simulink model "heli_master_2015b"  (R2015b)
settings: Solver=ode1  SolverMode=SingleTasking  StartTime=0.0  StopTime=inf  FixedStep=0.002  RelTol=1e-3
PostLoadFcn:
  | qc_set_target_type(getConfigSet(bdroot, 'QUARC Default Target Configuration'));
values from neighbouring files (symbols this model uses):
  K = P_predicted * C' * inv(C * P_predicted * C' + obj.W)    [ExtendedKalmanFilter.m]    (also in HighGainObserver.m = zeros(8, 2); StateFeedback.m = zeros(2, 6))
  lamb = block.ContStates.Data(3)    [BetterSimulation.m]    (also in FeedbackLinearization.m = x(3); dyn_ext_eps_meas.mat = [0 0 0 0 0 0 0 0 0 0 0 0 ... (30000 elements, 6000x5)]; e_-10_10_l_0_120_t_10.mat = [0 3.40359280049e-12 1.08295188827e-10 8.177826625e-10 3.426; e_-10_10_l_0_120_t_20.mat = [0 1.06295178385e-13 3.38915391498e-12 2.56636695446e-11 1.0)
  phi = block.ContStates.Data(1)    [BetterSimulation.m]    (also in FeedbackLinearization.m = x(1); dyn_ext_eps_meas.mat = [0 0 0 0 0 0 0 0 0 0 0 0 ... (18000 elements, 6000x3)]; e_-10_10_l_0_120_t_10.mat = [3.57789727367e-14 3.32260230971e-07 2.63920782562e-06 8.843; e_-10_10_l_0_120_t_20.mat = [3.52494450884e-15 1.04005854531e-08 8.29611824462e-08 2.791)
  R = diag(R_diag)    [compute_lqr_feedback.m]    (also in first_tvlqr_test.mat = [1  0; 0  1])
  vb = block.InputPort(2).Data    [BetterSimulation.m]    (also in analyze_eps_meas.m = [log_neg.signals(2).values; log_pos.signals(2).values]; dyn_ext_eps_meas.mat = [2.46662433384 2.46662437608 2.46662467016 2.46662546356 2.4; e_-10_10_l_0_120_t_10.mat = [3.03305943788 3.0306076999 3.02819113358 3.02581096907 3.02; e_-10_10_l_0_120_t_20.mat = [3.03305943788 3.0329822422 3.03290486178 3.03282733913 3.03)
  vf = block.InputPort(1).Data    [BetterSimulation.m]    (also in analyze_eps_meas.m = [log_neg.signals(1).values; log_pos.signals(1).values]; dyn_ext_eps_meas.mat = [2.46662433384 2.46662437608 2.46662467016 2.46662546356 2.4; e_-10_10_l_0_120_t_10.mat = [3.03305943788 3.03551133878 3.03792903521 3.04031223633 3.0; e_-10_10_l_0_120_t_20.mat = [3.03305943788 3.03313663866 3.03321405463 3.03329167331 3.0)
undefined symbols (not defined in the file or in its folder): HIL, qc_get_step_size
libraries: simulink_extras x25, quarc_library x4
(part 1 of 2)
settings Model: SimulationMode=external  ExtModeTrigDuration=120000  ExtModeTrigLevel=0.500000  Creator=Rchan  LastModifiedBy=robertph
settings SolverCC: PositivePriorityOrder=on
settings DataIOCC: SaveFormat=Array
settings OptimizationCC: ExpressionDepthLimit=2147483647  InitFltsAndDblsToZero=on
settings DebuggingCC: SaveWithParameterizedLinksMsg=none  UnderspecifiedInitializationDetection=Classic  MergeDetectMultiDrivingBlocksExec=none  SolverPrmCheckMsg=warning  MultiTaskDSMMsg=warning  FcnCallInpInsideContextMsg=EnableAllAsWarning  AllowSymbolicDim=on  StateNameClashWarn=warning
settings HardwareCC: ProdBitPerPointer=32  ProdLargestAtomicFloat=None  ProdIntDivRoundTo=Undefined  ProdEndianess=Unspecified  ProdWordSize=32  ProdHWDeviceType=32-bit Generic
settings RTWCC: SystemTargetFile=quarc_win64.tlc  TemplateMakefile=quarc_default_tmf  Description=QUARC Win64 Target
settings GRTTargetCC: ParMdlRefBuildCompliant=off  CompOptLevelCompliant=off  GeneratePreprocessorConditionals=Disable all  CombineOutputUpdateFcns=off  MatFileLogging=off  GRTInterface=on  UseToolchainInfoCompliant=off  ExtMode=on  ExtModeMexFile=quarc_comm
settings ConfigComp: CovModelRefEnable=Off  CovSFcnEnable=off

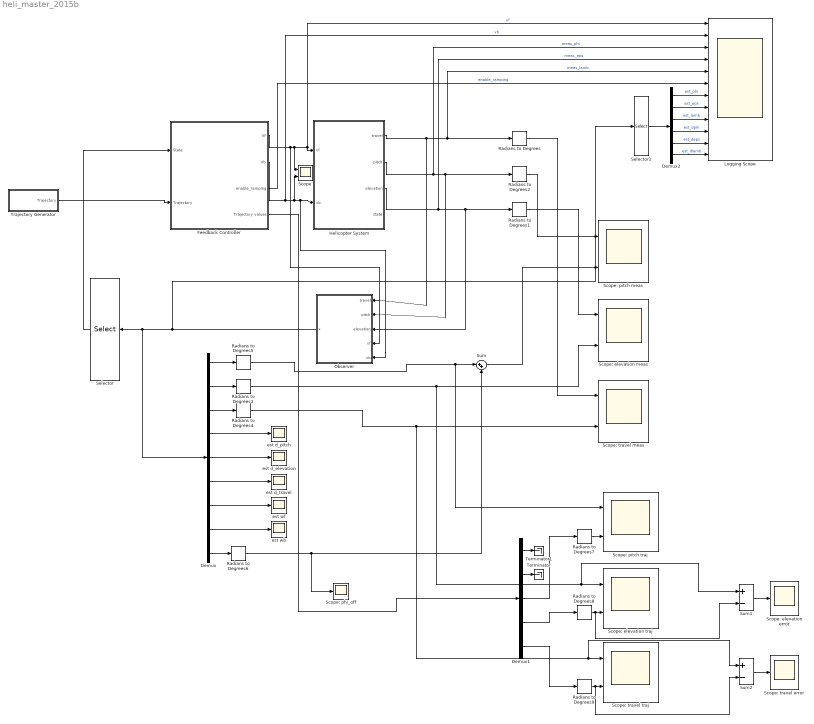
== system heli_master_2015b ==
  Demux : Demux  Outputs=9
  Demux1 : Demux  Outputs=5
  Demux2 : Demux  Outputs=6
  Feedback Controller : Subsystem
  Helicopter System : Subsystem  Variant=on  OverrideUsingVariant=HiL
  Logging Scope : Scope  NumInputPorts=12
  Observer : Subsystem
  Radians to Degrees{,1..9} (10 alike) : simulink_extras/Transformations/Radians to Degrees
  Scope : Scope  NumInputPorts=2
  Scope: elevation error : Scope
  Scope: elevation meas : Scope  NumInputPorts=2
  Scope: elevation traj : Scope  NumInputPorts=2
  Scope: phi_off : Scope
  Scope: pitch meas : Scope  NumInputPorts=2
  Scope: pitch traj : Scope  NumInputPorts=2
  Scope: travel error : Scope
  Scope: travel meas : Scope  NumInputPorts=2
  Scope: travel traj : Scope  NumInputPorts=2
  Selector : Selector  InputPortWidth=9  IndexOptions=Index vector (dialog)  Indices=[1 2 3 4 5 6 7 8]  OutputSizes=1
  Selector1 : Selector  InputPortWidth=9  IndexOptions=Index vector (dialog)  Indices=[1 2 3 4 5 6]  OutputSizes=1
  Sum : Sum  Inputs=|++
  Sum1 : Sum  Inputs=+-
  Sum2 : Sum  Inputs=+-
  Terminator : Terminator
  Terminator1 : Terminator
  Trajectory Generator : Subsystem
  est d_elevation : Scope
  est d_pitch : Scope
  est d_travel : Scope
  est wb : Scope
  est wf : Scope
  wires:
  Helicopter System/1(travel) -> Observer/1(travel), Logging Scope/5, Radians to Degrees/1  "meas_lamb"
  Helicopter System/3(elevation) -> Logging Scope/4, Observer/3(elevation), Radians to Degrees1/1  "meas_eps"
  Helicopter System/2(pitch) -> Logging Scope/3, Observer/2(pitch), Radians to Degrees2/1  "meas_phi"
  Radians to Degrees/1 -> Scope: travel meas/1
  Radians to Degrees2/1 -> Scope: pitch meas/1
  Radians to Degrees1/1 -> Scope: elevation meas/1
  Feedback Controller/2(Vb) -> Logging Scope/2, Scope/2, Observer/5(vb), Helicopter System/2(vb)  "vb"
  Feedback Controller/1(Vf) -> Observer/4(vf), Scope/1, Logging Scope/1, Helicopter System/1(vf)  "vf"
  Observer/1(x) -> Selector1/1, Selector/1, Demux/1
  Trajectory Generator/1(Trajectory) -> Feedback Controller/2(Trajectory)
  Demux/1 -> Radians to Degrees5/1
  Radians to Degrees3/1 -> Sum1/1, Scope: elevation traj/1, Scope: elevation meas/2
  Radians to Degrees4/1 -> Sum2/1, Scope: travel traj/1, Scope: travel meas/2
  Demux/2 -> Radians to Degrees3/1
  Demux/3 -> Radians to Degrees4/1
  Demux/4 -> est d_pitch/1
  Demux/5 -> est d_elevation/1
  Demux/6 -> est d_travel/1
  Demux/7 -> est wf/1
  Demux/8 -> est wb/1
  Demux/9 -> Radians to Degrees6/1
  Radians to Degrees5/1 -> Scope: pitch traj/1, Sum/1
  Sum/1 -> Scope: pitch meas/2
  Radians to Degrees6/1 -> Scope: phi_off/1, Sum/2
  Feedback Controller/3(enable_ramping) -> Logging Scope/6  "enable_ramping"
  Selector/1 -> Feedback Controller/1(State)
  Demux1/3 -> Radians to Degrees7/1
  Radians to Degrees7/1 -> Scope: pitch traj/2
  Radians to Degrees8/1 -> Sum1/2, Scope: elevation traj/2
  Radians to Degrees9/1 -> Sum2/2, Scope: travel traj/2
  Feedback Controller/4(Trajectory values) -> Demux1/1
  Demux1/4 -> Radians to Degrees8/1
  Demux1/5 -> Radians to Degrees9/1
  Demux1/2 -> Terminator/1
  Demux1/1 -> Terminator1/1
  Sum1/1 -> Scope: elevation error/1
  Sum2/1 -> Scope: travel error/1
  Selector1/1 -> Demux2/1
  Demux2/1 -> Logging Scope/7  "est_phi"
  Demux2/2 -> Logging Scope/8  "est_eps"
  Demux2/3 -> Logging Scope/9  "est_lamb"
  Demux2/4 -> Logging Scope/10  "est_dphi"
  Demux2/5 -> Logging Scope/11  "est_deps"
  Demux2/6 -> Logging Scope/12  "est_dlamb"

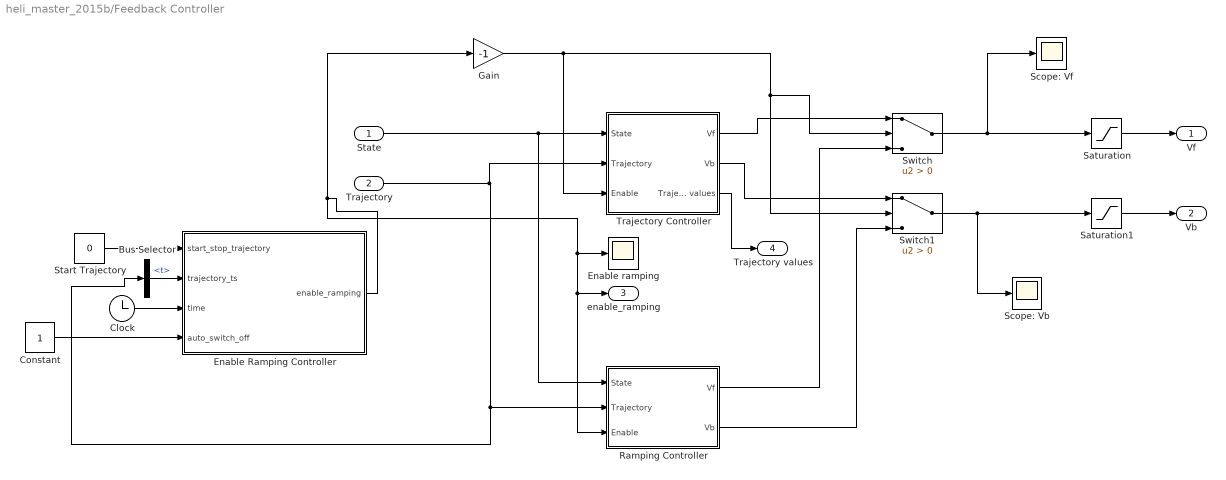
== system heli_master_2015b/Feedback Controller ==
  State : Inport
  Trajectory : Inport  Port=2
  Bus Selector : BusSelector  OutputSignals=t
  Clock : Clock
  Constant : Constant
  Enable Ramping Controller : MATLAB Function  TreatAsAtomicUnit=on
  Enable ramping : Scope
  Gain : Gain  Gain=-1
  Ramping Controller : Subsystem  mask(Ramping PID controller){ramp_period=0.1, deps_op=5, dlamb_op=10}
      mask prompts: ramp_period "Ramp period (s)"; deps_op "Elevation rate (deg/s)"; dlamb_op "Travel rate (deg/s)"
      mask help: Stabilizes an operating point, target is slowly ramped to set values.
  Saturation : Saturate  UpperLimit=5  LowerLimit=-5
  Saturation1 : Saturate  UpperLimit=5  LowerLimit=-5
  Scope: Vb : Scope
  Scope: Vf : Scope
  Start Trajectory : Constant  Value=0
  Switch : Switch  Criteria=u2 > Threshold
  Switch1 : Switch  Criteria=u2 > Threshold
  Trajectory Controller : Subsystem
  Vf : Outport
  Vb : Outport  Port=2
  enable_ramping : Outport  Port=3
  Trajectory values : Outport  Port=4
  wires:
  State/1 -> Ramping Controller/1(State), Trajectory Controller/1(State)
  Trajectory/1 -> Trajectory Controller/2(Trajectory), Bus Selector/1, Ramping Controller/2(Trajectory)
  Ramping Controller/1(Vf) -> Switch/3
  Ramping Controller/2(Vb) -> Switch1/3
  Start Trajectory/1 -> Enable Ramping Controller/1(start_stop_trajectory)
  Gain/1 -> Trajectory Controller/3(Enable), Switch1/2, Switch/2
  Switch/1 -> Saturation/1, Scope: Vf/1
  Switch1/1 -> Saturation1/1, Scope: Vb/1
  Trajectory Controller/1(Vf) -> Switch/1
  Trajectory Controller/2(Vb) -> Switch1/1
  Bus Selector/1 -> Enable Ramping Controller/2(trajectory_ts)  "<t>"
  Clock/1 -> Enable Ramping Controller/3(time)
  Saturation/1 -> Vf/1
  Saturation1/1 -> Vb/1
  Constant/1 -> Enable Ramping Controller/4(auto_switch_off)
  Enable Ramping Controller/1(enable_ramping) -> Enable ramping/1, enable_ramping/1, Ramping Controller/3(Enable), Gain/1
  Trajectory Controller/3(Trajectory values) -> Trajectory values/1

== system heli_master_2015b/Helicopter System ==
  note: 1) Add Subsystem or Model blocks as valid variant choices.
      | 2) You cannot connect blocks at this level. At simulation, connectivity is automatically
      | determined, based on the active variant and port name matching.
  vf : Inport
  vb : Inport  Port=2
  Helicopter Simulation : Subsystem  VariantControl=BetterSim  mask{ang0=[0, -20, 0], dang0=[0, 0, 0], w0=[0, 0]}
      mask prompts: ang0 "Pitch, Elevation, Travel (deg)"; dang0 "Angular velocities (deg/s)"; w0 "Rotor velocities"
      mask DialogControl DescTextVar Prompt: Simulates the helicopter system based on the equations of motion specified in system_f.m
  HiL : Subsystem  VariantControl=HiL
  Simple Simulation : Subsystem  VariantControl=SimpleSim
  Simulation with dynamic extension : Subsystem  VariantControl=DynamicExtensionSim
  travel : Outport
  pitch : Outport  Port=2
  elevation : Outport  Port=3
  state : Outport  Port=4

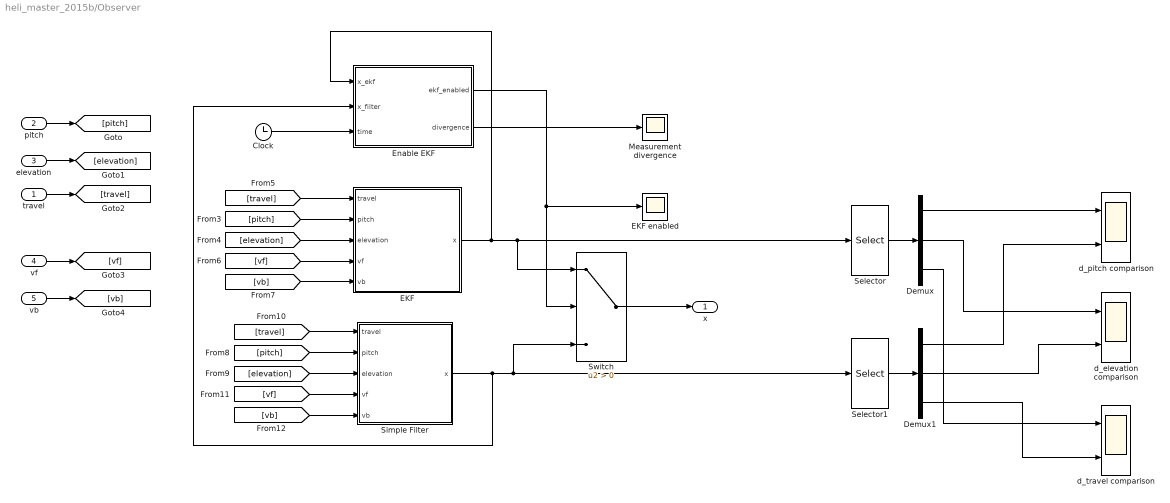
== system heli_master_2015b/Observer ==
  travel : Inport  PortDimensions=1
  pitch : Inport  Port=2  PortDimensions=1
  elevation : Inport  Port=3  PortDimensions=1
  vf : Inport  Port=4  PortDimensions=1
  vb : Inport  Port=5  PortDimensions=1
  Clock : Clock
  Demux : Demux  Outputs=3
  Demux1 : Demux  Outputs=3
  EKF : Subsystem  VariantControl=EKF
  EKF enabled : Scope
  Enable EKF : MATLAB Function  TreatAsAtomicUnit=on
  Measurement divergence : Scope
  Selector : Selector  InputPortWidth=9  IndexOptions=Index vector (dialog)  Indices=[4 5 6]  OutputSizes=1
  Selector1 : Selector  InputPortWidth=9  IndexOptions=Index vector (dialog)  Indices=[4 5 6]  OutputSizes=1
  Simple Filter : Subsystem  VariantControl=SimpleFilter
  Switch : Switch  Criteria=u2 > Threshold
  d_elevation comparison : Scope  NumInputPorts=2
  d_pitch comparison : Scope  NumInputPorts=2
  d_travel comparison : Scope  NumInputPorts=2
  x : Outport
  wires:
  Switch/1 -> x/1
  EKF/1(x) -> Enable EKF/1(x_ekf), Selector/1, Switch/1
  Simple Filter/1(x) -> Enable EKF/2(x_filter), Selector1/1, Switch/3
  Enable EKF/1(ekf_enabled) -> EKF enabled/1, Switch/2
  pitch/1 -> [pitch]
  vb/1 -> [vb]
  vf/1 -> [vf]
  travel/1 -> [travel]
  elevation/1 -> [elevation]
  [travel] -> EKF/1(travel)
  [elevation] -> EKF/3(elevation)
  [pitch] -> EKF/2(pitch)
  [vb] -> EKF/5(vb)
  [vf] -> EKF/4(vf)
  [travel] -> Simple Filter/1(travel)
  [elevation] -> Simple Filter/3(elevation)
  [pitch] -> Simple Filter/2(pitch)
  [vb] -> Simple Filter/5(vb)
  [vf] -> Simple Filter/4(vf)
  Clock/1 -> Enable EKF/3(time)
  Enable EKF/2(divergence) -> Measurement divergence/1
  Selector/1 -> Demux/1
  Selector1/1 -> Demux1/1
  Demux/1 -> d_pitch comparison/1
  Demux1/1 -> d_pitch comparison/2
  Demux/2 -> d_elevation comparison/1
  Demux1/2 -> d_elevation comparison/2
  Demux/3 -> d_travel comparison/1
  Demux1/3 -> d_travel comparison/2

== system heli_master_2015b/Trajectory Generator ==
  Bus Creator : BusCreator  Inputs=6
  Constant : Constant  Value=t
  Constant1 : Constant  Value=phi  VectorParams1D=off
  Constant2 : Constant  Value=eps  VectorParams1D=off
  Constant3 : Constant  Value=lamb  VectorParams1D=off
  Constant4 : Constant  Value=vf  VectorParams1D=off
  Constant5 : Constant  Value=vb  VectorParams1D=off
  Trajectory : Outport
  wires:
  Constant/1 -> Bus Creator/1  "t"
  Constant5/1 -> Bus Creator/6  "vb"
  Constant4/1 -> Bus Creator/5  "vf"
  Constant3/1 -> Bus Creator/4  "lamb"
  Constant2/1 -> Bus Creator/3  "eps"
  Constant1/1 -> Bus Creator/2  "phi"
  Bus Creator/1 -> Trajectory/1

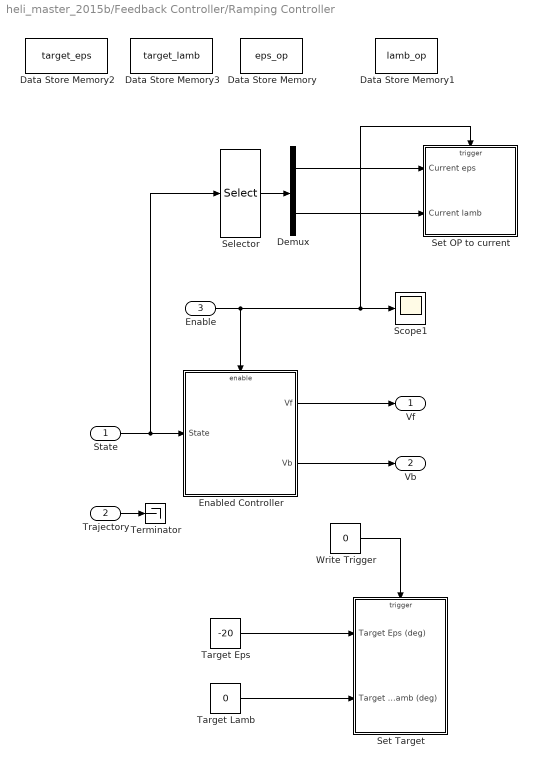
== system heli_master_2015b/Feedback Controller/Ramping Controller ==
  State : Inport
  Trajectory : Inport  Port=2
  Enable : Inport  Port=3
  Data Store Memory : DataStoreMemory  DataStoreName=eps_op  ReadBeforeWriteMsg=warning  WriteAfterWriteMsg=warning  WriteAfterReadMsg=warning  InitialValue=-29 / 180 * pi
  Data Store Memory1 : DataStoreMemory  DataStoreName=lamb_op  ReadBeforeWriteMsg=warning  WriteAfterWriteMsg=warning  WriteAfterReadMsg=warning
  Data Store Memory2 : DataStoreMemory  DataStoreName=target_eps  ReadBeforeWriteMsg=warning  WriteAfterWriteMsg=warning  WriteAfterReadMsg=warning  InitialValue=-29  OutDataTypeStr=double
  Data Store Memory3 : DataStoreMemory  DataStoreName=target_lamb  ReadBeforeWriteMsg=warning  WriteAfterWriteMsg=warning  WriteAfterReadMsg=warning  OutDataTypeStr=double
  Demux : Demux  Outputs=2
  Enabled Controller : Subsystem
  Scope1 : Scope
  Selector : Selector  InputPortWidth=8  IndexOptions=Index vector (dialog)  Indices=[2 3]  OutputSizes=1
  Set OP to current : Subsystem
  Set Target : Subsystem
  Target Eps : Constant  Value=-20
  Target Lamb : Constant  Value=0
  Terminator : Terminator
  Write Trigger : Constant  Value=0
  Vf : Outport
  Vb : Outport  Port=2
  wires:
  Enable/1 -> Scope1/1, Set OP to current/Trigger, Enabled Controller/Enable
  Demux/1 -> Set OP to current/1(Current eps)
  Demux/2 -> Set OP to current/2(Current lamb)
  State/1 -> Selector/1, Enabled Controller/1(State)
  Enabled Controller/2(Vb) -> Vb/1
  Enabled Controller/1(Vf) -> Vf/1
  Selector/1 -> Demux/1
  Target Lamb/1 -> Set Target/2(Target Lamb (deg))
  Target Eps/1 -> Set Target/1(Target Eps (deg))
  Write Trigger/1 -> Set Target/Trigger
  Trajectory/1 -> Terminator/1

== system heli_master_2015b/Feedback Controller/Trajectory Controller ==
  State : Inport
  Trajectory : Inport  Port=2
  Enable : Inport  Port=3
  Clock : Clock
  Data Store Memory : DataStoreMemory  DataStoreName=t0  ReadBeforeWriteMsg=warning  WriteAfterWriteMsg=warning  WriteAfterReadMsg=warning
  Data Store Read : DataStoreRead  Priority=10  DataStoreName=t0  SampleTime=0.002
  Enabled Controller : Subsystem
  Reset Time : Subsystem  Priority=0
  Sum : Sum  Inputs=-+|
  Vf : Outport
  Vb : Outport  Port=2
  Trajectory values : Outport  Port=3
  wires:
  Clock/1 -> Reset Time/1(Time), Sum/2
  Data Store Read/1 -> Sum/1
  Enabled Controller/1(Vf) -> Vf/1
  Enabled Controller/2(Vb) -> Vb/1
  Trajectory/1 -> Enabled Controller/3(Trajectory)
  State/1 -> Enabled Controller/2(State)
  Sum/1 -> Enabled Controller/1(Time)
  Enable/1 -> Enabled Controller/Enable, Reset Time/Trigger
  Enabled Controller/3(Trajectory values) -> Trajectory values/1

== system heli_master_2015b/Helicopter System/Helicopter Simulation ==
  vf : Inport
  vb : Inport  Port=2
  Level-2 MATLAB S-Function : M-S-Function  FunctionName=BetterSimulation  Parameters=ang0(1), ang0(2), ang0(3), dang0(1), dang0(2), dang0(3), w0(1), w0(2)
  Vector Concatenate : Concatenate  NumInputs=8
  d_elevation : Scope
  d_pitch : Scope
  d_travel : Scope
  dd_elevation : Scope
  dd_pitch : Scope
  dd_travel : Scope
  wb : Scope
  wf : Scope
  pitch : Outport
  elevation : Outport  Port=2
  travel : Outport  Port=3
  state : Outport  Port=4
  wires:
  vf/1 -> Level-2 MATLAB S-Function/1
  vb/1 -> Level-2 MATLAB S-Function/2
  Level-2 MATLAB S-Function/1 -> Vector Concatenate/1, pitch/1
  Level-2 MATLAB S-Function/3 -> Vector Concatenate/3, travel/1
  Level-2 MATLAB S-Function/2 -> Vector Concatenate/2, elevation/1
  Level-2 MATLAB S-Function/4 -> Vector Concatenate/4, d_pitch/1  "sim_dphi"
  Level-2 MATLAB S-Function/8 -> Vector Concatenate/8, wb/1  "sim_wb"
  Level-2 MATLAB S-Function/7 -> Vector Concatenate/7, wf/1  "sim_wf"
  Level-2 MATLAB S-Function/6 -> Vector Concatenate/6, d_travel/1  "sim_dlamb"
  Level-2 MATLAB S-Function/5 -> Vector Concatenate/5, d_elevation/1  "sim_deps"
  Level-2 MATLAB S-Function/10 -> dd_elevation/1  "sim_ddeps"
  Level-2 MATLAB S-Function/11 -> dd_travel/1  "sim_ddlamb"
  Level-2 MATLAB S-Function/9 -> dd_pitch/1  "sim_ddphi"
  Vector Concatenate/1 -> state/1

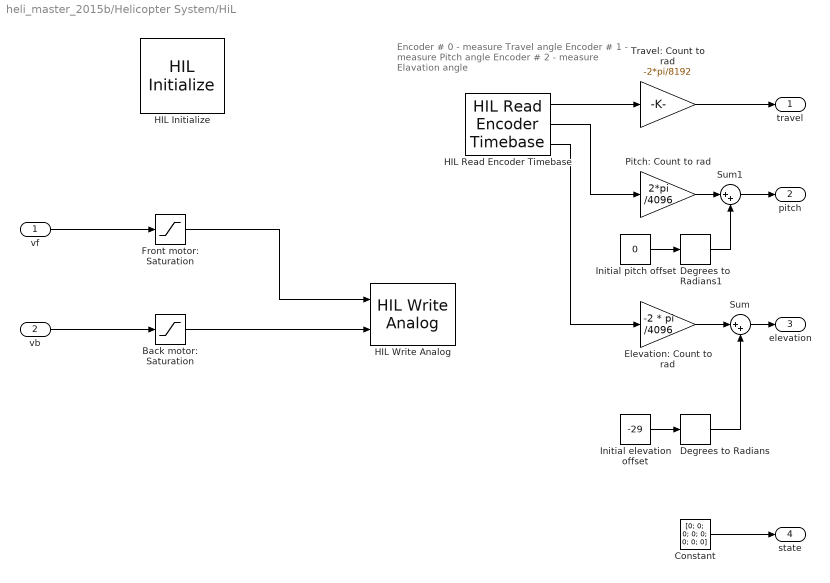
== system heli_master_2015b/Helicopter System/HiL ==
  note: Encoder # 0 - measure Travel angle
      | Encoder # 1 - measure Pitch angle
      | Encoder # 2 - measure Elavation angle
  vf : Inport
  vb : Inport  Port=2
  Back motor: Saturation : Saturate  UpperLimit=5  LowerLimit=-5
  Constant : Constant  Value=[0; 0; 0; 0; 0; 0; 0; 0]
  Degrees to Radians : simulink_extras/Transformations/Degrees to Radians
  Degrees to Radians1 : simulink_extras/Transformations/Degrees to Radians
  Elevation: Count to rad : Gain  Gain=-2 * pi /4096
  Front motor: Saturation : Saturate  UpperLimit=5  LowerLimit=-5
  HIL Initialize : quarc_library/Data Acquisition/Generic/Configuration/HIL Initialize  Priority=-99  object_name=HIL-1  board_type=q8_usb  board_number=0  board_options=update_rate=normal;decimation=1  exclusive=off  active=off  hardware_clocks=[0:2]  clock_modes=[]  initial_clock_frequencies=[]  set_clock_params_at_start=off  set_clock_params_at_switch_in=off  set_clock_frequencies_at_start=off  set_clock_frequencies_at_switch_in=off  analog_input_channels=[0:7]  analog_input_maximums=10  analog_input_minimums=-10  set_analog_input_params_at_start=on  set_analog_input_params_at_switch_in=off  analog_output_channels=[0:7]  analog_output_maximums=10  analog_output_minimums=-10  initial_analog_outputs=[0]  final_analog_outputs=[0]  watchdog_analog_outputs=0  set_analog_output_params_at_start=on  set_analog_output_params_at_switch_in=off  set_analog_outputs_at_start=on  set_analog_outputs_at_switch_in=off  set_analog_outputs_at_terminate=on  set_analog_outputs_at_switch_out=off  set_analog_outputs_on_watchdog=off  digital_input_channels=[]  digital_output_channels=[]  digital_output_configuration=[]  initial_digital_outputs=[1]  final_digital_outputs=[1]  watchdog_digital_outputs=[1]  set_digital_output_params_at_start=off  set_digital_output_params_at_switch_in=off  set_digital_outputs_at_start=on  set_digital_outputs_at_switch_in=off  set_digital_outputs_at_terminate=on  set_digital_outputs_at_switch_out=off  set_digital_outputs_on_watchdog=off  encoder_channels=[0:7]  quadrature=[4]  encoder_filter_frequency=[]  initial_encoder_counts=[0]  set_encoder_params_at_start=on  set_encoder_params_at_switch_in=off  set_encoder_counts_at_start=on  set_encoder_counts_at_switch_in=off  pwm_channels=[0:7]  pwm_modes=0  pwm_frequency=99.532799999999995e6/4095  pwm_configuration=[0]  pwm_alignment=[0]  pwm_polarity=[1]  pwm_leading_deadband=[0]  pwm_trailing_deadband=[0]  initial_pwm_outputs=[0]  final_pwm_outputs=[0]  watchdog_pwm_outputs=[0]  set_pwm_params_at_start=on  set_pwm_params_at_switch_in=off  set_pwm_outputs_at_start=on  set_pwm_outputs_at_switch_in=off  set_pwm_outputs_at_terminate=on  set_pwm_outputs_at_switch_out=off  set_pwm_outputs_on_watchdog=off  other_output_channels=[]  initial_other_outputs=[]  final_other_outputs=[]  watchdog_other_outputs=[]  set_other_outputs_at_start=off  set_other_outputs_at_switch_in=off  set_other_outputs_at_terminate=off  set_other_outputs_at_switch_out=off  set_other_outputs_on_watchdog=off
  HIL Read Encoder Timebase : quarc_library/Data Acquisition/Generic/Timebases/HIL Read Encoder Timebase  object_name=HIL-1  clock=0  channels=[0:2]  samples_in_buffer=max(ceil(1/qc_get_step_size), 1)  active=on  vector_output=off  data_type_mode=Inherit via back propagation  data_type=double
  HIL Write Analog : quarc_library/Data Acquisition/Generic/Immediate I//O/HIL Write Analog  object_name=HIL-1  channels=[0:1]  sample_time=-1  active=off  vector_input=off
  Initial elevation offset : Constant  Value=-29
  Initial pitch offset : Constant  Value=0
  Pitch: Count to rad : Gain  Gain=2*pi /4096
  Sum : Sum  Inputs=|++
  Sum1 : Sum  Inputs=|++
  Travel: Count to rad : Gain  Gain=-2*pi/8192
  travel : Outport
  pitch : Outport  Port=2
  elevation : Outport  Port=3
  state : Outport  Port=4
  wires:
  vf/1 -> Front motor: Saturation/1
  vb/1 -> Back motor: Saturation/1
  Back motor: Saturation/1 -> HIL Write Analog/2
  HIL Read Encoder Timebase/2 -> Pitch: Count to rad/1
  HIL Read Encoder Timebase/1 -> Travel: Count to rad/1
  Front motor: Saturation/1 -> HIL Write Analog/1
  HIL Read Encoder Timebase/3 -> Elevation: Count to rad/1
  Travel: Count to rad/1 -> travel/1
  Elevation: Count to rad/1 -> Sum/1
  Sum/1 -> elevation/1
  Initial elevation offset/1 -> Degrees to Radians/1
  Degrees to Radians/1 -> Sum/2
  Pitch: Count to rad/1 -> Sum1/1
  Sum1/1 -> pitch/1
  Initial pitch offset/1 -> Degrees to Radians1/1
  Degrees to Radians1/1 -> Sum1/2
  Constant/1 -> state/1

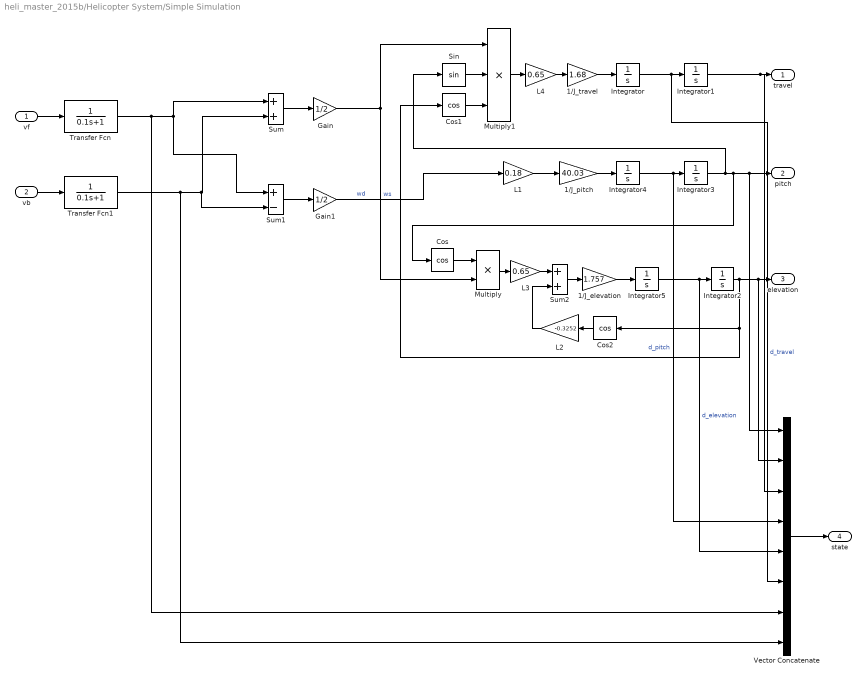
== system heli_master_2015b/Helicopter System/Simple Simulation ==
  vf : Inport
  vb : Inport  Port=2
  1/J_elevation : Gain  Gain=1.757
  1/J_pitch : Gain  Gain=40.03
  1/J_travel : Gain  Gain=1.68
  Cos : Trigonometry  Operator=cos
  Cos1 : Trigonometry  Operator=cos
  Cos2 : Trigonometry  Operator=cos
  Gain : Gain  Gain=1/2
  Gain1 : Gain  Gain=1/2
  Integrator : Integrator
  Integrator1 : Integrator  LimitOutput=on  UpperSaturationLimit=2.1  LowerSaturationLimit=-2.1
  Integrator2 : Integrator  LimitOutput=on  UpperSaturationLimit=1.22  LowerSaturationLimit=-1.22
  Integrator3 : Integrator  LimitOutput=on  UpperSaturationLimit=1.4  LowerSaturationLimit=-1.4
  Integrator4 : Integrator
  Integrator5 : Integrator
  L1 : Gain  Gain=0.18
  L2 : Gain  Gain=-0.3252
  L3 : Gain  Gain=0.65
  L4 : Gain  Gain=0.65
  Multiply : Product
  Multiply1 : Product  Inputs=3
  Sin : Trigonometry
  Sum : Sum
  Sum1 : Sum  Inputs=+-
  Sum2 : Sum
  Transfer Fcn : TransferFcn  Denominator=[0.1 1]
  Transfer Fcn1 : TransferFcn  Denominator=[0.1 1]
  Vector Concatenate : Concatenate  NumInputs=8
  travel : Outport
  pitch : Outport  Port=2
  elevation : Outport  Port=3
  state : Outport  Port=4
  wires:
  Integrator/1 -> Vector Concatenate/6, Integrator1/1  "d_travel"
  Integrator1/1 -> Vector Concatenate/3, travel/1
  Integrator3/1 -> Sin/1, Cos/1, Vector Concatenate/1, pitch/1
  Integrator4/1 -> Vector Concatenate/4, Integrator3/1  "d_pitch"
  Integrator2/1 -> Cos2/1, Cos1/1, Vector Concatenate/2, elevation/1
  Integrator5/1 -> Vector Concatenate/5, Integrator2/1  "d_elevation"
  Sum/1 -> Gain/1
  Sum1/1 -> Gain1/1
  1/J_pitch/1 -> Integrator4/1
  L1/1 -> 1/J_pitch/1
  Gain1/1 -> L1/1  "wd"
  Cos/1 -> Multiply/1
  Gain/1 -> Multiply1/1, Multiply/2  "ws"
  1/J_elevation/1 -> Integrator5/1
  1/J_travel/1 -> Integrator/1
  Multiply/1 -> L3/1
  Multiply1/1 -> L4/1
  L4/1 -> 1/J_travel/1
  Sin/1 -> Multiply1/2
  Cos1/1 -> Multiply1/3
  Sum2/1 -> 1/J_elevation/1
  L3/1 -> Sum2/1
  L2/1 -> Sum2/2
  Cos2/1 -> L2/1
  vf/1 -> Transfer Fcn/1
  vb/1 -> Transfer Fcn1/1
  Transfer Fcn/1 -> Vector Concatenate/7, Sum1/1, Sum/1
  Transfer Fcn1/1 -> Vector Concatenate/8, Sum1/2, Sum/2
  Vector Concatenate/1 -> state/1

== system heli_master_2015b/Helicopter System/Simulation with dynamic extension ==
  vf : Inport
  vb : Inport  Port=2
  MATLAB System : MATLABSystem  System=DynamicExtensionSim  x0=zeros(8, 1)  SimulateUsing=Code generation
      mask Type: DynamicExtensionSim
      mask Display:
      | disp('DynamicExtensionSim');
      | port_label('input',1,'uf');
      | port_label('input',2,'ub');
      | port_label('output',1,'x');
  pitch : Outport
  elevation : Outport  Port=2
  travel : Outport  Port=3
  state : Outport  Port=4

== system heli_master_2015b/Observer/EKF ==
  travel : Inport
  pitch : Inport  Port=2
  elevation : Inport  Port=3
  vf : Inport  Port=4
  vb : Inport  Port=5
  Estimator : Subsystem  mask(Extended Kalman Filter){x0=[ 0; deg2rad( -29 ); 0; 0; 0; 0; 0; 0; deg2rad(6) ], P_diag=[1, 1, 1, 1, 1, 1, 1, 1, 1], N_diag=[ 100, 100 ], W_diag=[ 0.0001, 0.00001, 0.00001 ], step_width=0.002}
      mask help: Estimates system state based on measured system inputs, outputs, and knowledge about associated noise parameters.
      mask DialogControl Control2 Prompt: x0:
      mask DialogControl Control3 Prompt: diag(P):
      mask DialogControl Control4 Prompt: diag(N):
      mask DialogControl Control5 Prompt: diag(W):
      mask DialogControl Control6 Prompt: step width:
      mask Display:
      | disp('Extended Kalman Filter')
      | port_label('output', 1, 'State Estimate')
      | port_label('input', 1, 'Measurement')
      | port_label('input', 2, 'Control')
  Unit Delay : UnitDelay  InitialCondition=[0, 0]  SampleTime=-1
  Vector Concatenate : Concatenate  NumInputs=3
  Vector Concatenate1 : Concatenate
  x : Outport
  wires:
  Estimator/1(State Estimate) -> x/1
  Vector Concatenate/1 -> Estimator/1(Measurement)
  travel/1 -> Vector Concatenate/3
  elevation/1 -> Vector Concatenate/2
  pitch/1 -> Vector Concatenate/1
  vf/1 -> Vector Concatenate1/1
  vb/1 -> Vector Concatenate1/2
  Vector Concatenate1/1 -> Unit Delay/1
  Unit Delay/1 -> Estimator/2(Control)

== system heli_master_2015b/Observer/Simple Filter ==
  travel : Inport
  pitch : Inport  Port=2
  elevation : Inport  Port=3
  vf : Inport  Port=4
  vb : Inport  Port=5
  Constant : Constant  Value=6
  Degrees to Radians : simulink_extras/Transformations/Degrees to Radians
  Sum : Sum  Inputs=|+-
  Transfer Fcn : TransferFcn  Denominator=[0.01 1]
  Transfer Fcn1 : TransferFcn  Denominator=[0.01 1]
  Travel: Transfer Fcn : TransferFcn  Numerator=[50 0]  Denominator=[1 50]
  Travel: Transfer Fcn1 : TransferFcn  Numerator=[50 0]  Denominator=[1 50]
  Travel: Transfer Fcn2 : TransferFcn  Numerator=[50 0]  Denominator=[1 50]
  Vector Concatenate : Concatenate  NumInputs=9
  x : Outport
  wires:
  pitch/1 -> Sum/1, Travel: Transfer Fcn/1
  elevation/1 -> Vector Concatenate/2, Travel: Transfer Fcn1/1
  travel/1 -> Vector Concatenate/3, Travel: Transfer Fcn2/1
  Vector Concatenate/1 -> x/1
  Travel: Transfer Fcn/1 -> Vector Concatenate/4
  Travel: Transfer Fcn1/1 -> Vector Concatenate/5
  Travel: Transfer Fcn2/1 -> Vector Concatenate/6
  Transfer Fcn/1 -> Vector Concatenate/7
  vf/1 -> Transfer Fcn/1
  Transfer Fcn1/1 -> Vector Concatenate/8
  vb/1 -> Transfer Fcn1/1
  Constant/1 -> Degrees to Radians/1
  Sum/1 -> Vector Concatenate/1
  Degrees to Radians/1 -> Sum/2, Vector Concatenate/9

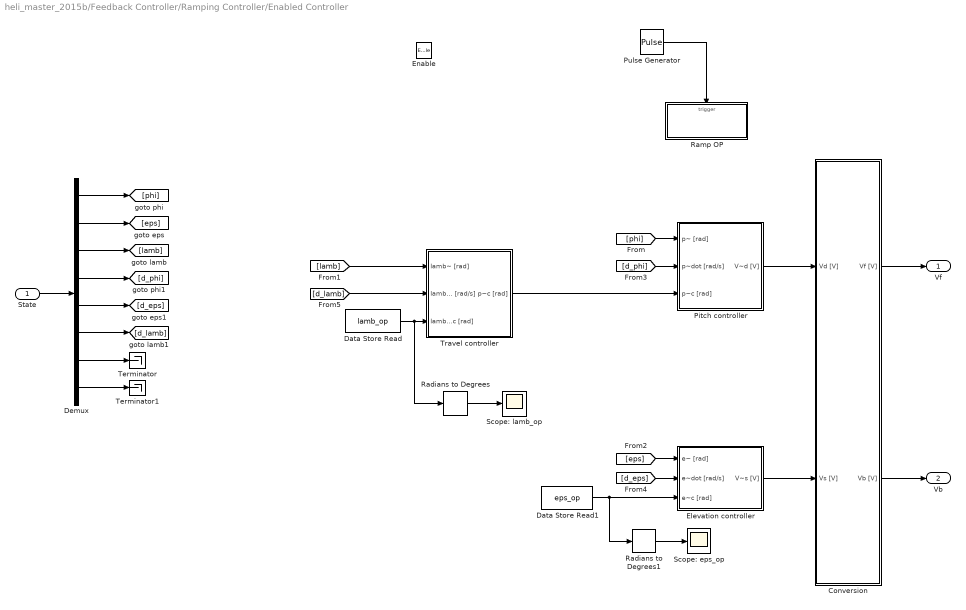
== system heli_master_2015b/Feedback Controller/Ramping Controller/Enabled Controller ==
  State : Inport
  Enable : EnablePort  StatesWhenEnabling=reset
  Conversion : Subsystem
  Data Store Read : DataStoreRead  DataStoreName=lamb_op  SampleTime=0.002
  Data Store Read1 : DataStoreRead  DataStoreName=eps_op  SampleTime=0.002
  Demux : Demux  Outputs=8
  Elevation controller : Subsystem
  Pitch controller : Subsystem
  Pulse Generator : DiscretePulseGenerator  PulseType=Time based  Period=ramp_period  PulseWidth=50  SampleTime=0.002
  Radians to Degrees : simulink_extras/Transformations/Radians to Degrees
  Radians to Degrees1 : simulink_extras/Transformations/Radians to Degrees
  Ramp OP : Subsystem
  Scope: eps_op : Scope
  Scope: lamb_op : Scope
  Terminator : Terminator
  Terminator1 : Terminator
  Travel controller : Subsystem
  Vf : Outport
  Vb : Outport  Port=2
  wires:
  State/1 -> Demux/1
  Demux/1 -> [phi]
  Demux/2 -> [eps]
  Demux/3 -> [lamb]
  Demux/4 -> [d_phi]
  Demux/5 -> [d_eps]
  Demux/6 -> [d_lamb]
  Conversion/2(Vb [V]) -> Vb/1
  Conversion/1(Vf [V]) -> Vf/1
  Elevation controller/1(V~s [V]) -> Conversion/2(Vs [V])
  Travel controller/1(p~c [rad]) -> Pitch controller/3(p~c [rad])
  [phi] -> Pitch controller/1(p~ [rad])
  [eps] -> Elevation controller/1(e~ [rad])
  [lamb] -> Travel controller/1(lamb~ [rad])
  [d_phi] -> Pitch controller/2(p~dot [rad/s])
  [d_eps] -> Elevation controller/2(e~dot [rad/s])
  [d_lamb] -> Travel controller/2(lamb~dot [rad/s])
  Data Store Read/1 -> Radians to Degrees/1, Travel controller/3(lamb~c [rad])
  Data Store Read1/1 -> Radians to Degrees1/1, Elevation controller/3(e~c [rad])
  Pulse Generator/1 -> Ramp OP/Trigger
  Radians to Degrees/1 -> Scope: lamb_op/1
  Radians to Degrees1/1 -> Scope: eps_op/1
  Pitch controller/1(V~d [V]) -> Conversion/1(Vd [V])
  Demux/7 -> Terminator/1
  Demux/8 -> Terminator1/1

== system heli_master_2015b/Feedback Controller/Ramping Controller/Set OP to current ==
  Current eps : Inport
  Current lamb : Inport  Port=2
  Trigger : TriggerPort  PortDimensions=1
  Data Store Write : DataStoreWrite  DataStoreName=eps_op
  Data Store Write1 : DataStoreWrite  DataStoreName=lamb_op
  Data Store Write2 : DataStoreWrite  DataStoreName=target_eps
  Data Store Write3 : DataStoreWrite  DataStoreName=target_lamb
  Radians to Degrees : simulink_extras/Transformations/Radians to Degrees
  Radians to Degrees1 : simulink_extras/Transformations/Radians to Degrees
  wires:
  Current eps/1 -> Radians to Degrees/1, Data Store Write/1
  Current lamb/1 -> Radians to Degrees1/1, Data Store Write1/1
  Radians to Degrees/1 -> Data Store Write2/1
  Radians to Degrees1/1 -> Data Store Write3/1

== system heli_master_2015b/Feedback Controller/Ramping Controller/Set Target ==
  Target Eps (deg) : Inport
  Target Lamb (deg) : Inport  Port=2
  Trigger : TriggerPort  PortDimensions=1
  Data Store Write : DataStoreWrite  DataStoreName=target_eps
  Data Store Write1 : DataStoreWrite  DataStoreName=target_lamb
  wires:
  Target Eps (deg)/1 -> Data Store Write/1
  Target Lamb (deg)/1 -> Data Store Write1/1

== system heli_master_2015b/Feedback Controller/Trajectory Controller/Enabled Controller ==
  Time : Inport
  State : Inport  Port=2
  Trajectory : Inport  Port=3
  Enable : EnablePort  StatesWhenEnabling=reset
  Bus Selector : BusSelector  OutputSignals=t,phi,eps,lamb,vf,vb
  Demux : Demux  Outputs=2
  Evaluate Trajectory : MATLAB Function  TreatAsAtomicUnit=on
  Trajectory Controller Variants : Subsystem  Variant=on  OverrideUsingVariant=CascadePid
  Trajectory Time : Scope
  Vf : Outport
  Vb : Outport  Port=2
  Trajectory values : Outport  Port=3
  wires:
  Bus Selector/4 -> Evaluate Trajectory/4(traj_lamb), Trajectory Controller Variants/6(lamb_d)  "<lamb>"
  Trajectory/1 -> Bus Selector/1
  Bus Selector/1 -> Evaluate Trajectory/1(traj_t), Trajectory Controller Variants/3(t_d)  "<t>"
  Bus Selector/6 -> Evaluate Trajectory/6(traj_vb), Trajectory Controller Variants/8(vb_d)  "<vb>"
  Bus Selector/2 -> Evaluate Trajectory/2(traj_phi), Trajectory Controller Variants/4(phi_d)  "<phi>"
  Bus Selector/3 -> Evaluate Trajectory/3(traj_eps), Trajectory Controller Variants/5(eps_d)  "<eps>"
  Bus Selector/5 -> Evaluate Trajectory/5(traj_vf), Trajectory Controller Variants/7(vf_d)  "<vf>"
  State/1 -> Trajectory Controller Variants/2(x)
  Trajectory Controller Variants/1(u) -> Demux/1
  Demux/1 -> Vf/1
  Demux/2 -> Vb/1
  Time/1 -> Evaluate Trajectory/7(t), Trajectory Time/1, Trajectory Controller Variants/1(t)
  Evaluate Trajectory/1(vals) -> Trajectory values/1

== system heli_master_2015b/Feedback Controller/Trajectory Controller/Reset Time ==
  Time : Inport
  Trigger : TriggerPort  PortDimensions=1
  Data Store Write : DataStoreWrite  DataStoreName=t0
  wires:
  Time/1 -> Data Store Write/1

== system heli_master_2015b/Observer/EKF/Estimator ==
  Measurement : Inport
  Control : Inport  Port=2
  MATLAB Function : MATLAB Function  TreatAsAtomicUnit=on
  N_diag : Constant  Value=N_diag
  P_diag : Constant  Value=P_diag
  W_diag : Constant  Value=W_diag
  step_width : Constant  Value=step_width
  x0 : Constant  Value=x0
  State Estimate : Outport
  wires:
  MATLAB Function/1(x) -> State Estimate/1
  Measurement/1 -> MATLAB Function/1(y)
  Control/1 -> MATLAB Function/2(u)
  x0/1 -> MATLAB Function/3(x0)
  step_width/1 -> MATLAB Function/7(step_width)
  W_diag/1 -> MATLAB Function/6(W_diag)
  N_diag/1 -> MATLAB Function/5(N_diag)
  P_diag/1 -> MATLAB Function/4(P_diag)

== system heli_master_2015b/Feedback Controller/Ramping Controller/Enabled Controller/Conversion ==
  Vd [V] : Inport
  Vs [V] : Inport  Port=2
  Add : Sum
  Back gain : Gain  Gain=0.5
  Front gain : Gain  Gain=0.5
  Subtract : Sum  Inputs=+-
  Vf [V] : Outport
  Vb [V] : Outport  Port=2
  wires:
  Vd [V]/1 -> Subtract/2, Add/1
  Vs [V]/1 -> Subtract/1, Add/2
  Subtract/1 -> Back gain/1
  Back gain/1 -> Vb [V]/1
  Add/1 -> Front gain/1
  Front gain/1 -> Vf [V]/1

== system heli_master_2015b/Feedback Controller/Ramping Controller/Enabled Controller/Elevation controller ==
  e~ [rad] : Inport
  e~dot [rad/s] : Inport  Port=2
  e~c [rad] : Inport  Port=3
  Elevation controller : Subsystem
  Sum : Sum  Inputs=-+  SaturateOnIntegerOverflow=on  InputSameDT=on  OutDataTypeStr=Inherit: Same as first input
  V~s [V] : Outport  InitialOutput=0
  wires:
  Sum/1 -> Elevation controller/1(e~ [rad])
  Elevation controller/1(V~_s [V]) -> V~s [V]/1
  e~ [rad]/1 -> Sum/1
  e~dot [rad/s]/1 -> Elevation controller/2(e~_dot [rad/s])
  e~c [rad]/1 -> Sum/2

== system heli_master_2015b/Feedback Controller/Ramping Controller/Enabled Controller/Pitch controller ==
  p~ [rad] : Inport
  p~dot [rad/s] : Inport  Port=2
  p~c [rad] : Inport  Port=3
  Integrator : Integrator  LimitOutput=on
  Kd : Gain  Gain=3.5
  Ki : Gain  Gain=0.5
  Kp : Gain  Gain=8
  Saturation : Saturate  UpperLimit=10  LowerLimit=-10
  Sum : Sum  Inputs=+-
  Sum1 : Sum  Inputs=++-
  V~d [V] : Outport  InitialOutput=0
  wires:
  p~c [rad]/1 -> Sum/1
  p~ [rad]/1 -> Sum/2
  Sum/1 -> Ki/1, Kp/1
  p~dot [rad/s]/1 -> Kd/1
  Kp/1 -> Sum1/1
  Sum1/1 -> Saturation/1
  Saturation/1 -> V~d [V]/1
  Kd/1 -> Sum1/3
  Ki/1 -> Integrator/1
  Integrator/1 -> Sum1/2

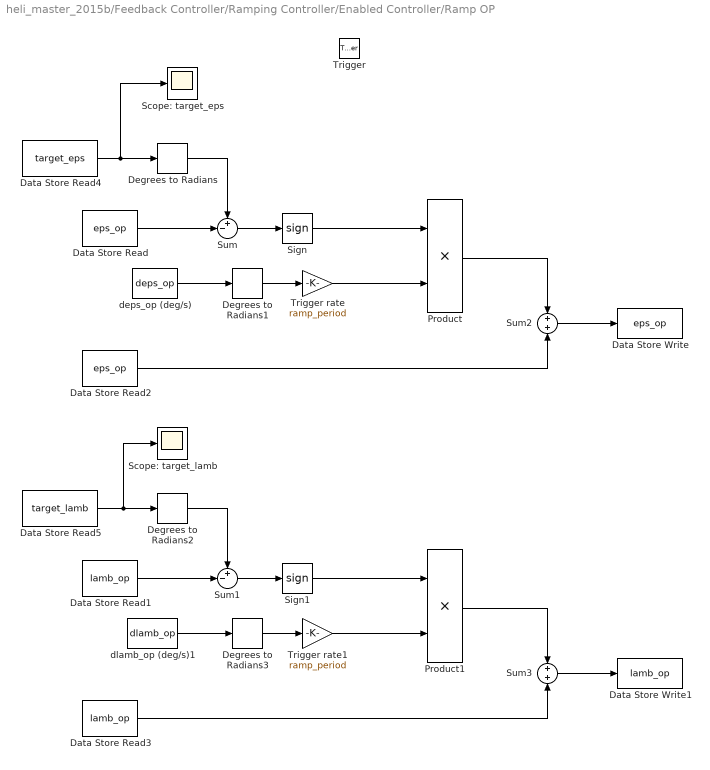
== system heli_master_2015b/Feedback Controller/Ramping Controller/Enabled Controller/Ramp OP ==
  Trigger : TriggerPort  PortDimensions=1
  Data Store Read : DataStoreRead  DataStoreName=eps_op
  Data Store Read1 : DataStoreRead  DataStoreName=lamb_op
  Data Store Read2 : DataStoreRead  DataStoreName=eps_op
  Data Store Read3 : DataStoreRead  DataStoreName=lamb_op
  Data Store Read4 : DataStoreRead  DataStoreName=target_eps
  Data Store Read5 : DataStoreRead  DataStoreName=target_lamb
  Data Store Write : DataStoreWrite  DataStoreName=eps_op
  Data Store Write1 : DataStoreWrite  DataStoreName=lamb_op
  Degrees to Radians{,1..3} (4 alike) : simulink_extras/Transformations/Degrees to Radians
  Product : Product
  Product1 : Product
  Scope: target_eps : Scope
  Scope: target_lamb : Scope
  Sign : Signum
  Sign1 : Signum
  Sum : Sum  Inputs=+-|
  Sum1 : Sum  Inputs=+-|
  Sum2 : Sum  Inputs=+|+
  Sum3 : Sum  Inputs=+|+
  Trigger rate : Gain  Gain=ramp_period
  Trigger rate1 : Gain  Gain=ramp_period
  deps_op (deg/s) : Constant  Value=deps_op
  dlamb_op (deg/s)1 : Constant  Value=dlamb_op
  wires:
  Data Store Read4/1 -> Scope: target_eps/1, Degrees to Radians/1
  Data Store Read/1 -> Sum/2
  Degrees to Radians/1 -> Sum/1
  Sum/1 -> Sign/1
  Sign/1 -> Product/1
  deps_op (deg/s)/1 -> Degrees to Radians1/1
  Degrees to Radians1/1 -> Trigger rate/1
  Trigger rate/1 -> Product/2
  Data Store Read5/1 -> Scope: target_lamb/1, Degrees to Radians2/1
  Data Store Read1/1 -> Sum1/2
  Degrees to Radians2/1 -> Sum1/1
  Sum1/1 -> Sign1/1
  Sign1/1 -> Product1/1
  dlamb_op (deg/s)1/1 -> Degrees to Radians3/1
  Degrees to Radians3/1 -> Trigger rate1/1
  Trigger rate1/1 -> Product1/2
  Product/1 -> Sum2/1
  Data Store Read2/1 -> Sum2/2
  Sum2/1 -> Data Store Write/1
  Product1/1 -> Sum3/1
  Data Store Read3/1 -> Sum3/2
  Sum3/1 -> Data Store Write1/1

== system heli_master_2015b/Feedback Controller/Ramping Controller/Enabled Controller/Travel controller ==
  lamb~ [rad] : Inport
  lamb~dot [rad/s] : Inport  Port=2
  lamb~c [rad] : Inport  Port=3
  Integrator : Integrator  LimitOutput=on
  Kd : Gain  Gain=1.3
  Ki : Gain  Gain=0.1
  Kp : Gain  Gain=0.8
  Saturation : Saturate  UpperLimit=20  LowerLimit=-20
  Sum : Sum  Inputs=+-
  Sum1 : Sum  Inputs=++-
  p~c [rad] : Outport  InitialOutput=0
  wires:
  lamb~c [rad]/1 -> Sum/1
  lamb~ [rad]/1 -> Sum/2
  Sum/1 -> Ki/1, Kp/1
  lamb~dot [rad/s]/1 -> Kd/1
  Kp/1 -> Sum1/1
  Saturation/1 -> p~c [rad]/1
  Kd/1 -> Sum1/3
  Ki/1 -> Integrator/1
  Integrator/1 -> Sum1/2
  Sum1/1 -> Saturation/1

== system heli_master_2015b/Feedback Controller/Trajectory Controller/Enabled Controller/Trajectory Controller Variants ==
  note: 1) Add Subsystem or Model blocks as valid variant choices.
      | 2) You cannot connect blocks at this level. At simulation, connectivity is automatically
      | determined, based on the active variant and port name matching.
  t : Inport
  x : Inport  Port=2  PortDimensions=8
  t_d : Inport  Port=3
  phi_d : Inport  Port=4
  eps_d : Inport  Port=5
  lamb_d : Inport  Port=6
  vf_d : Inport  Port=7
  vb_d : Inport  Port=8
  Ad hoc PID : Subsystem  VariantControl=AdHocPID
  CascadePid : Subsystem  VariantControl=CascadePid
  DynamicExtension : Subsystem  VariantControl=DynamicExtension
  Gain Scheduling PID : Subsystem  VariantControl=GainSchedulingPid
  Joystick PID : Subsystem  VariantControl=JoystickPID
  StateFeedback : Subsystem  VariantControl=StateFeedback
  TimeVariantLQR : Subsystem  VariantControl=TimeVariantLQR
  TimeVariantLQRI : Subsystem  VariantControl=TimeVariantLQRI
  u : Outport

== system heli_master_2015b/Feedback Controller/Ramping Controller/Enabled Controller/Elevation controller/Elevation controller ==
  e~ [rad] : Inport
  e~_dot [rad/s] : Inport  Port=2
  Integrator : Integrator  LimitOutput=on
  K_ed : Gain  Gain=20  SaturateOnIntegerOverflow=on  OutDataTypeStr=Inherit: Same as input  ParamDataTypeStr=Inherit: Same as input
  K_ei : Gain  Gain=20  SaturateOnIntegerOverflow=on  OutDataTypeStr=Inherit: Same as input  ParamDataTypeStr=Inherit: Same as input
  K_ep : Gain  Gain=30  SaturateOnIntegerOverflow=on  OutDataTypeStr=Inherit: Same as input  ParamDataTypeStr=Inherit: Same as input
  Sum : Sum  Inputs=++-  SaturateOnIntegerOverflow=on  InputSameDT=on  OutDataTypeStr=Inherit: Same as first input
  V~_s [V] : Outport  InitialOutput=0
  wires:
  K_ei/1 -> Integrator/1
  Integrator/1 -> Sum/1
  Sum/1 -> V~_s [V]/1
  e~_dot [rad/s]/1 -> K_ed/1
  K_ed/1 -> Sum/3
  K_ep/1 -> Sum/2
  e~ [rad]/1 -> K_ep/1, K_ei/1

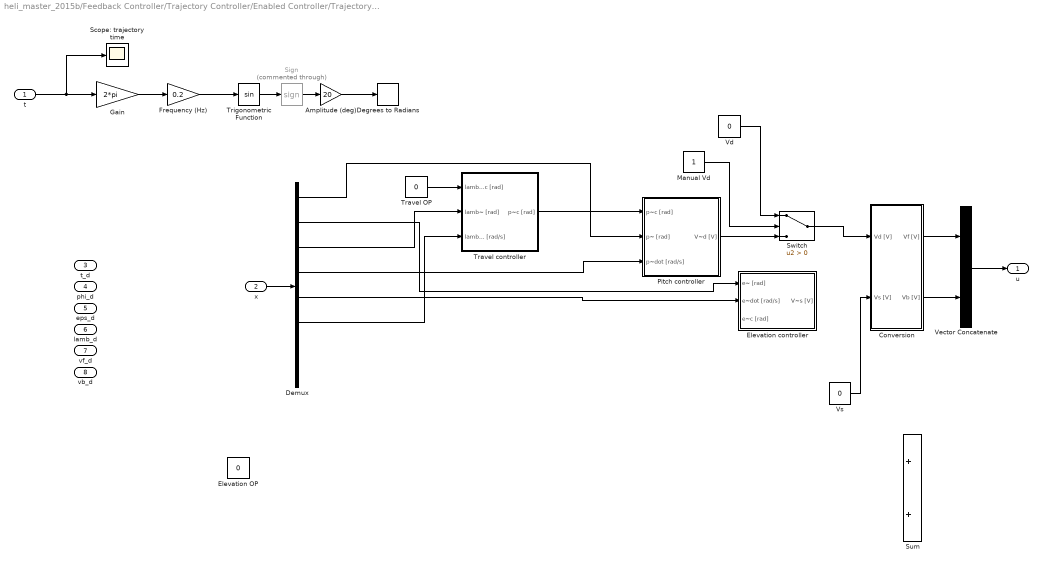
== system heli_master_2015b/Feedback Controller/Trajectory Controller/Enabled Controller/Trajectory Controller Variants/Ad hoc PID ==
  t : Inport
  x : Inport  Port=2
  t_d : Inport  Port=3
  phi_d : Inport  Port=4
  eps_d : Inport  Port=5
  lamb_d : Inport  Port=6
  vf_d : Inport  Port=7
  vb_d : Inport  Port=8
  Amplitude (deg) : Gain  Gain=20
  Conversion : Subsystem
  Degrees to Radians : simulink_extras/Transformations/Degrees to Radians
  Demux : Demux  Outputs=8
  Elevation OP : Constant  Value=0
  Elevation controller : Subsystem
  Frequency (Hz) : Gain  Gain=0.2
  Gain : Gain  Gain=2*pi
  Manual Vd : Constant
  Pitch controller : Subsystem
  Scope: trajectory time : Scope
  Sign : Signum  Commented=through
  Sum : Sum
  Switch : Switch  Criteria=u2 > Threshold
  Travel OP : Constant  Value=0
  Travel controller : Subsystem
  Trigonometric Function : Trigonometry
  Vd : Constant  Value=0
  Vector Concatenate : Concatenate
  Vs : Constant  Value=0
  u : Outport
  wires:
  Conversion/1(Vf [V]) -> Vector Concatenate/1
  Conversion/2(Vb [V]) -> Vector Concatenate/2
  x/1 -> Demux/1
  Demux/1 -> Pitch controller/2(p~ [rad])
  Demux/2 -> Elevation controller/1(e~ [rad])
  Demux/3 -> Travel controller/2(lamb~ [rad])
  Demux/4 -> Pitch controller/3(p~dot [rad/s])
  Demux/5 -> Elevation controller/2(e~dot [rad/s])
  Demux/6 -> Travel controller/3(lamb~dot [rad/s])
  Vector Concatenate/1 -> u/1
  t/1 -> Scope: trajectory time/1, Gain/1
  Gain/1 -> Frequency (Hz)/1
  Frequency (Hz)/1 -> Trigonometric Function/1
  Trigonometric Function/1 -> Sign/1
  Pitch controller/1(V~d [V]) -> Switch/3
  Manual Vd/1 -> Switch/2
  Switch/1 -> Conversion/1(Vd [V])
  Sign/1 -> Amplitude (deg)/1
  Amplitude (deg)/1 -> Degrees to Radians/1
  Travel controller/1(p~c [rad]) -> Pitch controller/1(p~c [rad])
  Travel OP/1 -> Travel controller/1(lamb~c [rad])
  Vd/1 -> Switch/1
  Vs/1 -> Conversion/2(Vs [V])

== system heli_master_2015b/Feedback Controller/Trajectory Controller/Enabled Controller/Trajectory Controller Variants/CascadePid ==
  t : Inport
  x : Inport  Port=2
  t_d : Inport  Port=3
  phi_d : Inport  Port=4
  eps_d : Inport  Port=5
  lamb_d : Inport  Port=6
  vf_d : Inport  Port=7
  vb_d : Inport  Port=8
  MATLAB System : MATLABSystem  System=CascadePid  elevation_pid_gains=[15, 0.1, 7]  travel_pitch_pid_gains=[2.5 0.05, 3]  pitch_vd_pid_gains=[4, 0.1, 2]  k_rotor=[ 0, 0 ]  feed_forward=on  rotor_speed_control=off  SimulateUsing=Code generation
      mask Type: CascadePid
      mask Display:
      | disp('CascadePid');
      | port_label('input',1,'Time');
      | port_label('input',2,'State');
      | port_label('input',3,'Traj Time');
      | port_label('input',4,'Traj Phi');
      | port_label('input',5,'Traj Eps');
      | port_label('input',6,'Traj Lamb');
      | port_label('input',7,'Traj Vf');
      | port_label('input',8,'Traj Vb');
      | port_label('output',1,'Control');
      | port_label('output',2,'Debug');
  Scope : Scope
  u : Outport
  wires:
  MATLAB System/1 -> u/1
  vb_d/1 -> MATLAB System/8
  vf_d/1 -> MATLAB System/7
  lamb_d/1 -> MATLAB System/6
  eps_d/1 -> MATLAB System/5
  phi_d/1 -> MATLAB System/4
  t_d/1 -> MATLAB System/3
  x/1 -> MATLAB System/2
  t/1 -> MATLAB System/1
  MATLAB System/2 -> Scope/1

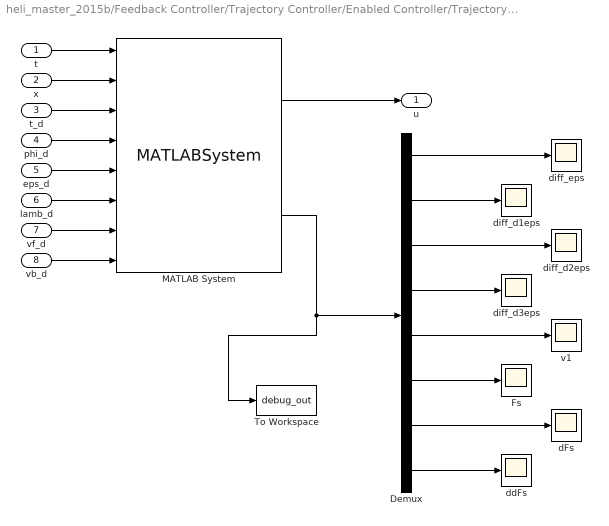
== system heli_master_2015b/Feedback Controller/Trajectory Controller/Enabled Controller/Trajectory Controller Variants/DynamicExtension ==
  t : Inport
  x : Inport  Port=2
  t_d : Inport  Port=3
  phi_d : Inport  Port=4
  eps_d : Inport  Port=5
  lamb_d : Inport  Port=6
  vf_d : Inport  Port=7
  vb_d : Inport  Port=8
  Demux : Demux  Outputs=8
  Fs : Scope
  MATLAB System : MATLABSystem  System=DynamicExtension  k_eps=[ 16, 32, 24, 8 ]  k_lamb=[ 16, 32, 24, 8 ]  x780=[ 0.7; 0 ]  step_width=0.002  SimulateUsing=Code generation
      mask Type: DynamicExtension
      mask Display:
      | disp('DynamicExtension');
      | port_label('input',1,'Time');
      | port_label('input',2,'State');
      | port_label('input',3,'Traj Time');
      | port_label('input',4,'Traj Phi');
      | port_label('input',5,'Traj Eps');
      | port_label('input',6,'Traj Lamb');
      | port_label('input',7,'Traj Vf');
      | port_label('input',8,'Traj Vb');
      | port_label('output',1,'Control');
      | port_label('output',2,'Debug');
  To Workspace : ToWorkspace  VariableName=debug_out  SaveFormat=Structure With Time  SampleTime=-1
  dFs : Scope
  ddFs : Scope
  diff_d1eps : Scope
  diff_d2eps : Scope
  diff_d3eps : Scope
  diff_eps : Scope
  v1 : Scope
  u : Outport
  wires:
  MATLAB System/1 -> u/1
  vb_d/1 -> MATLAB System/8
  vf_d/1 -> MATLAB System/7
  lamb_d/1 -> MATLAB System/6
  eps_d/1 -> MATLAB System/5
  phi_d/1 -> MATLAB System/4
  t_d/1 -> MATLAB System/3
  x/1 -> MATLAB System/2
  t/1 -> MATLAB System/1
  MATLAB System/2 -> To Workspace/1, Demux/1
  Demux/1 -> diff_eps/1
  Demux/2 -> diff_d1eps/1
  Demux/3 -> diff_d2eps/1
  Demux/4 -> diff_d3eps/1
  Demux/5 -> v1/1
  Demux/6 -> Fs/1
  Demux/7 -> dFs/1
  Demux/8 -> ddFs/1

== system heli_master_2015b/Feedback Controller/Trajectory Controller/Enabled Controller/Trajectory Controller Variants/Gain Scheduling PID ==
  t : Inport
  x : Inport  Port=2
  t_d : Inport  Port=3
  phi_d : Inport  Port=4
  eps_d : Inport  Port=5
  lamb_d : Inport  Port=6
  vf_d : Inport  Port=7
  vb_d : Inport  Port=8
  MATLAB System : MATLABSystem  System=GainSchedulingPid  elevation_levels=[ -20, -10, 0, 10, 20 ]  elevation_pid_gains=[ 15, 0.1, 7 ]  travel_pitch_pid_gains=[ 10, 0, 10; 5, 0, 5; 2, 0, 2; 2, 0, 2; 2.5, 0, 2.5 ]  pitch_vd_pid_gains=[ 4, 0.1, 2 ]  k_rotor=[ 0, 0 ]  feed_forward=on  rotor_speed_control=off  SimulateUsing=Code generation
      mask Type: GainSchedulingPid
      mask Display:
      | disp('GainSchedulingPid');
      | port_label('input',1,'Time');
      | port_label('input',2,'State');
      | port_label('input',3,'Traj Time');
      | port_label('input',4,'Traj Phi');
      | port_label('input',5,'Traj Eps');
      | port_label('input',6,'Traj Lamb');
      | port_label('input',7,'Traj Vf');
      | port_label('input',8,'Traj Vb');
      | port_label('output',1,'Control');
      | port_label('output',2,'Debug');
  Scope : Scope
  u : Outport
  wires:
  MATLAB System/1 -> u/1
  vb_d/1 -> MATLAB System/8
  vf_d/1 -> MATLAB System/7
  lamb_d/1 -> MATLAB System/6
  eps_d/1 -> MATLAB System/5
  phi_d/1 -> MATLAB System/4
  t_d/1 -> MATLAB System/3
  x/1 -> MATLAB System/2
  t/1 -> MATLAB System/1
  MATLAB System/2 -> Scope/1

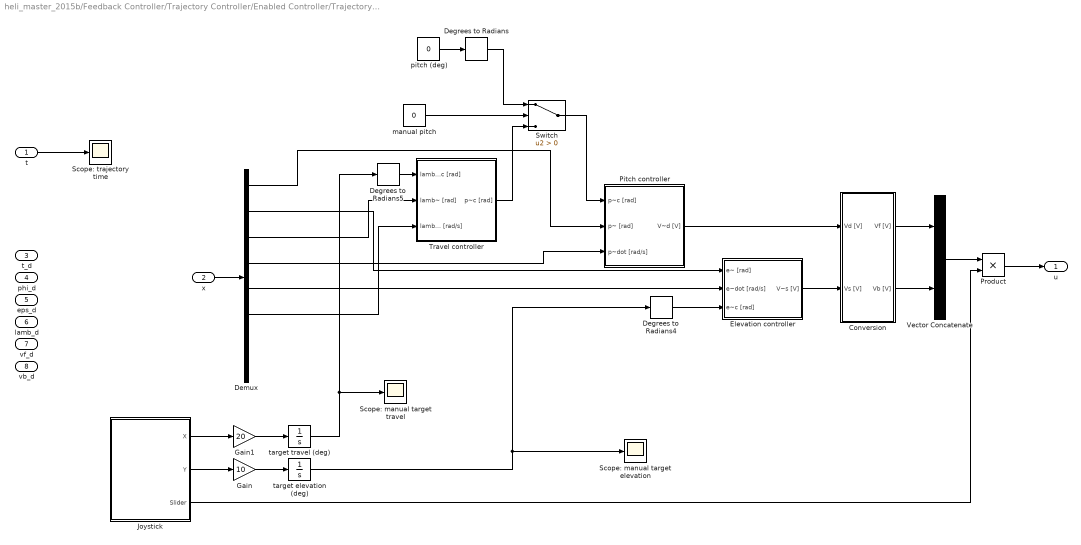
== system heli_master_2015b/Feedback Controller/Trajectory Controller/Enabled Controller/Trajectory Controller Variants/Joystick PID ==
  t : Inport
  x : Inport  Port=2
  t_d : Inport  Port=3
  phi_d : Inport  Port=4
  eps_d : Inport  Port=5
  lamb_d : Inport  Port=6
  vf_d : Inport  Port=7
  vb_d : Inport  Port=8
  Conversion : Subsystem
  Degrees to Radians : simulink_extras/Transformations/Degrees to Radians
  Degrees to Radians4 : simulink_extras/Transformations/Degrees to Radians
  Degrees to Radians5 : simulink_extras/Transformations/Degrees to Radians
  Demux : Demux  Outputs=8
  Elevation controller : Subsystem
  Gain : Gain  Gain=10
  Gain1 : Gain  Gain=20
  Joystick : Subsystem
  Pitch controller : Subsystem
  Product : Product
  Scope: manual target elevation : Scope
  Scope: manual target travel : Scope
  Scope: trajectory time : Scope
  Switch : Switch  Criteria=u2 > Threshold
  Travel controller : Subsystem
  Vector Concatenate : Concatenate
  manual pitch : Constant  Value=0
  pitch (deg) : Constant  Value=0
  target elevation (deg) : Integrator  InitialCondition=-29  LimitOutput=on  UpperSaturationLimit=30  LowerSaturationLimit=-30
  target travel (deg) : Integrator  LimitOutput=on  UpperSaturationLimit=180  LowerSaturationLimit=-180
  u : Outport
  wires:
  Conversion/1(Vf [V]) -> Vector Concatenate/1
  Conversion/2(Vb [V]) -> Vector Concatenate/2
  Elevation controller/1(V~s [V]) -> Conversion/2(Vs [V])
  Pitch controller/1(V~d [V]) -> Conversion/1(Vd [V])
  x/1 -> Demux/1
  Demux/1 -> Pitch controller/2(p~ [rad])
  Demux/2 -> Elevation controller/1(e~ [rad])
  Demux/3 -> Travel controller/2(lamb~ [rad])
  Demux/4 -> Pitch controller/3(p~dot [rad/s])
  Demux/5 -> Elevation controller/2(e~dot [rad/s])
  Demux/6 -> Travel controller/3(lamb~dot [rad/s])
  Degrees to Radians5/1 -> Travel controller/1(lamb~c [rad])
  Degrees to Radians4/1 -> Elevation controller/3(e~c [rad])
  Joystick/2(Y) -> Gain/1
  Gain/1 -> target elevation (deg)/1
  Joystick/1(X) -> Gain1/1
  Gain1/1 -> target travel (deg)/1
  target elevation (deg)/1 -> Scope: manual target elevation/1, Degrees to Radians4/1
  target travel (deg)/1 -> Scope: manual target travel/1, Degrees to Radians5/1
  Vector Concatenate/1 -> Product/1
  Product/1 -> u/1
  Joystick/3(Slider) -> Product/2
  t/1 -> Scope: trajectory time/1
  Switch/1 -> Pitch controller/1(p~c [rad])
  Travel controller/1(p~c [rad]) -> Switch/3
  pitch (deg)/1 -> Degrees to Radians/1
  Degrees to Radians/1 -> Switch/1
  manual pitch/1 -> Switch/2

== system heli_master_2015b/Feedback Controller/Trajectory Controller/Enabled Controller/Trajectory Controller Variants/StateFeedback ==
  t : Inport
  x : Inport  Port=2
  t_d : Inport  Port=3
  phi_d : Inport  Port=4
  eps_d : Inport  Port=5
  lamb_d : Inport  Port=6
  vf_d : Inport  Port=7
  vb_d : Inport  Port=8
  MATLAB System : MATLABSystem  System=StateFeedback  K=K  SimulateUsing=Code generation
      mask Type: StateFeedback
      mask Display:
      | disp('StateFeedback');
      | port_label('input',1,'Time');
      | port_label('input',2,'State');
      | port_label('input',3,'Traj Time');
      | port_label('input',4,'Traj Phi');
      | port_label('input',5,'Traj Eps');
      | port_label('input',6,'Traj Lamb');
      | port_label('input',7,'Traj Vf');
      | port_label('input',8,'Traj Vb');
      | port_label('output',1,'Control');
      | port_label('output',2,'Debug');
  u : Outport
  wires:
  MATLAB System/1 -> u/1
  vb_d/1 -> MATLAB System/8
  vf_d/1 -> MATLAB System/7
  lamb_d/1 -> MATLAB System/6
  eps_d/1 -> MATLAB System/5
  phi_d/1 -> MATLAB System/4
  t_d/1 -> MATLAB System/3
  x/1 -> MATLAB System/2
  t/1 -> MATLAB System/1
